simulink model "variables"  (R2020a)
settings: Solver=VariableStepAuto  StartTime=0.0  StopTime=300  RelTol=1e-3
values from neighbouring files (symbols this model uses):
  denGcs = [1 1.984]    [variables.mat]
  denGcz = [1 -0.137518063444]    [variables.mat]
  denGs = [1 0.1 0]    [variables.mat]
  K = 17    [variables.mat]
  Kc = 4.59510193011    [variables.mat]
  numGcs = [1 0.1963]    [variables.mat]
  numGcz = [1 -0.914664715652]    [variables.mat]
  numGs = [0 0 0.1]    [variables.mat]
  T = 1    [variables.mat]
settings Model: Creator=filip  LastModifiedBy=filip

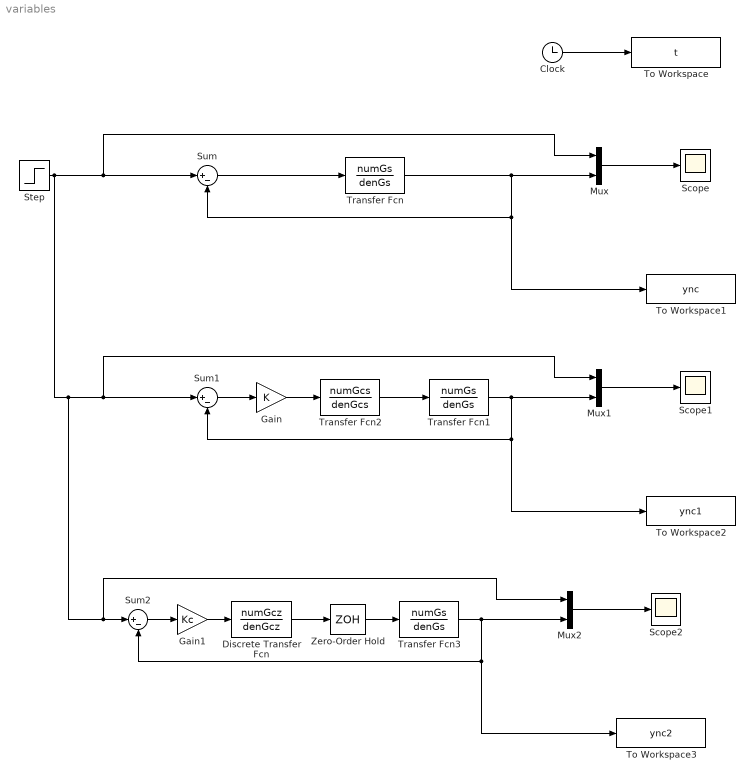
== system variables ==
  Clock : Clock
  Discrete Transfer Fcn : DiscreteTransferFcn  Numerator=numGcz  Denominator=denGcz  SampleTime=T
  Gain : Gain  Gain=K
  Gain1 : Gain  Gain=Kc
  Mux : Mux  Inputs=2
  Mux1 : Mux  Inputs=2
  Mux2 : Mux  Inputs=2
  Scope : Scope
  Scope1 : Scope
  Scope2 : Scope
  Step : Step  Time=0  SampleTime=0
  Sum : Sum  Inputs=|+-
  Sum1 : Sum  Inputs=|+-
  Sum2 : Sum  Inputs=|+-
  To Workspace : ToWorkspace  VariableName=t  SampleTime=-1
  To Workspace1 : ToWorkspace  VariableName=ync  SampleTime=-1
  To Workspace2 : ToWorkspace  VariableName=ync1  SampleTime=-1
  To Workspace3 : ToWorkspace  VariableName=ync2  SampleTime=-1
  Transfer Fcn : TransferFcn  Numerator=numGs  Denominator=denGs
  Transfer Fcn1 : TransferFcn  Numerator=numGs  Denominator=denGs
  Transfer Fcn2 : TransferFcn  Numerator=numGcs  Denominator=denGcs
  Transfer Fcn3 : TransferFcn  Numerator=numGs  Denominator=denGs
  Zero-Order Hold : ZeroOrderHold  SampleTime=T
  wires:
  Transfer Fcn/1 -> To Workspace1/1, Sum/2, Mux/2
  Mux/1 -> Scope/1
  Sum/1 -> Transfer Fcn/1
  Clock/1 -> To Workspace/1
  Transfer Fcn1/1 -> To Workspace2/1, Sum1/2, Mux1/2
  Mux1/1 -> Scope1/1
  Transfer Fcn2/1 -> Transfer Fcn1/1
  Gain/1 -> Transfer Fcn2/1
  Sum1/1 -> Gain/1
  Gain1/1 -> Discrete Transfer Fcn/1
  Zero-Order Hold/1 -> Transfer Fcn3/1
  Step/1 -> Sum1/1, Mux1/1, Mux2/1, Sum2/1, Mux/1, Sum/1
  Mux2/1 -> Scope2/1
  Transfer Fcn3/1 -> Mux2/2, To Workspace3/1, Sum2/2
  Sum2/1 -> Gain1/1
  Discrete Transfer Fcn/1 -> Zero-Order Hold/1
